simulink model "SIM_EXO_DAL"  (R2021b)
settings: Solver=VariableStepAuto  StartTime=0.0  StopTime=60  FixedStep=0.0001  RelTol=1e-4
undefined symbols (not defined in the file): b, dq, q, X, Y, Z
libraries: sm_lib x47, nesl_utility x7
(part 25 of 25)

== matlab function SIM_EXO_DAL/PD+g(DIN)/MATLAB Function ==
  data: H input; ts input; b input; Kp output; Kd output
function [Kp, Kd] = ganancias(H,ts,b)
Kp = zeros(6,1);
Kd = zeros(6,1);

wn = 6/ts;
be = 5.02e-6;
for i = 1:6
    Kp(i) = H(i,i)*(wn^2);
    Kd(i) = H(i,i)*(2*(wn^2))-b(i)-be;

    if Kp(i) < 0 
        Kp(i) = 0;
    end
    if Kd(i) < 0 
        Kd(i) = 0;
    end
end
